simulink model "Fuzzy_BLDC"  (R2023a)
settings: Solver=ode1  StartTime=0.0  StopTime=50  FixedStep=0.1  RelTol=1e-3
values from neighbouring files (symbols this model uses):
  command_values = 0:6    [GenerateLUT_Fuzzy.m]
  error_pitch_values = -90:5:90    [GenerateLUT_Fuzzy.m]
  error_yaw_values = -180:5:180    [GenerateLUT_Fuzzy.m]
  fuzzy_lut_pitch = zeros(length(error_pitch_values), length(var_error_pitch_values), length(command_values), 2)    [GenerateLUT_Fuzzy.m]
  fuzzy_lut_yaw = zeros(length(error_yaw_values), length(var_error_yaw_values), length(command_values), 2)    [GenerateLUT_Fuzzy.m]
  var_error_pitch_values = -30:5:30    [GenerateLUT_Fuzzy.m]
  var_error_yaw_values = -50:5:50    [GenerateLUT_Fuzzy.m]
settings Model: Creator=yafhers  LastModifiedBy=yafhers
settings OptimizationCC: BlockReduction=off  ConditionallyExecuteInputs=off  DefaultParameterBehavior=Inlined  EnhancedBackFolding=on  PassReuseOutputArgsAs=Individual arguments  ZeroExternalMemoryAtStartup=off  ZeroInternalMemoryAtStartup=off  OptimizeBlockOrder=speed  DifferentSizesBufferReuse=on  OptimizationCustomize=off  EfficientTunableParamExpr=on
settings DebuggingCC: ParameterTunabilityLossMsg=error
settings SFSimCC: MATLABDynamicMemAlloc=off  SimTargetLang=C++
settings RTWCC: Description=Embedded Coder  SystemTargetFile=ert.tlc  TemplateMakefile=ert_default_tmf
settings CodeAppCC: ForceParamTrailComments=on  IgnoreCustomStorageClasses=off  OperatorAnnotations=on  SimulinkDataObjDesc=on  SFDataObjDesc=on  InsertBlockDesc=on
settings ERTTargetCC: TargetLangStandard=C99 (ISO)  GenerateSampleERTMain=on  InlinedParameterPlacement=NonHierarchical  ERTCustomFileTemplate=example_file_process.tlc

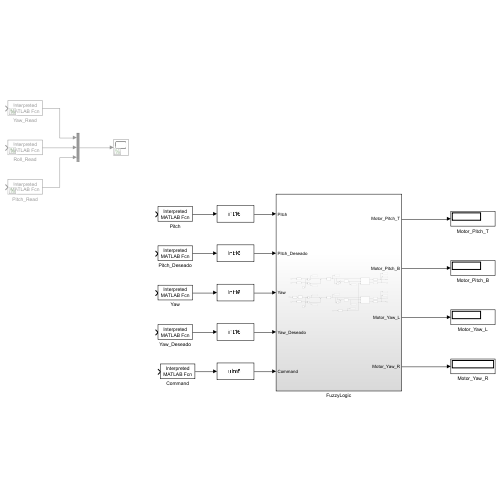
[thumbnail: Simulink's stored preview of the top-level diagram]
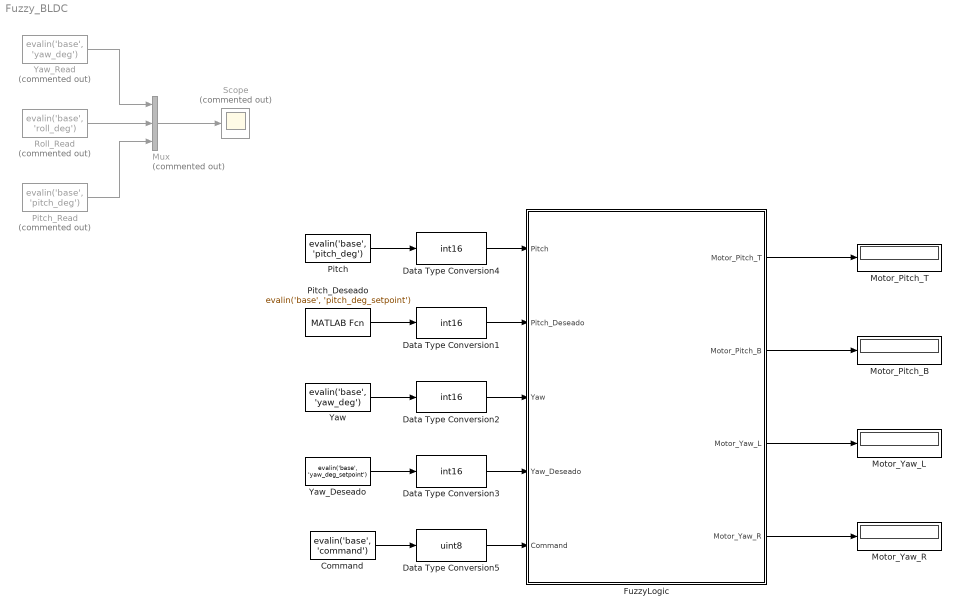
== system Fuzzy_BLDC ==
  Command : MATLABFcn  MATLABFcn=evalin('base', 'command')  OutputDimensions=1
  Data Type Conversion{1..4} (4 alike) : DataTypeConversion  OutDataTypeStr=int16  SaturateOnIntegerOverflow=off  RndMeth=Floor
  Data Type Conversion5 : DataTypeConversion  OutDataTypeStr=uint8  SaturateOnIntegerOverflow=off  RndMeth=Floor
  FuzzyLogic : Subsystem
  Motor_Pitch_B : Display
  Motor_Pitch_T : Display
  Motor_Yaw_L : Display
  Motor_Yaw_R : Display
  Mux : Mux  Commented=on  Inputs=3
  Pitch : MATLABFcn  MATLABFcn=evalin('base', 'pitch_deg')  OutputDimensions=1
  Pitch_Deseado : MATLABFcn  MATLABFcn=evalin('base', 'pitch_deg_setpoint')  OutputDimensions=1
  Pitch_Read : MATLABFcn  Commented=on  MATLABFcn=evalin('base', 'pitch_deg')  OutputDimensions=1  OutputSignalType=real
  Roll_Read : MATLABFcn  Commented=on  MATLABFcn=evalin('base', 'roll_deg')  OutputDimensions=1  OutputSignalType=real
  Scope : Scope  Commented=on
  Yaw : MATLABFcn  MATLABFcn=evalin('base', 'yaw_deg')  OutputDimensions=1
  Yaw_Deseado : MATLABFcn  MATLABFcn=evalin('base', 'yaw_deg_setpoint')  OutputDimensions=1
  Yaw_Read : MATLABFcn  Commented=on  MATLABFcn=evalin('base', 'yaw_deg')  OutputDimensions=1  OutputSignalType=real
  wires:
  Roll_Read/1 -> Mux/2
  Yaw_Read/1 -> Mux/1
  Pitch_Read/1 -> Mux/3
  Mux/1 -> Scope/1
  FuzzyLogic/2(Motor_Pitch_B) -> Motor_Pitch_B/1
  FuzzyLogic/1(Motor_Pitch_T) -> Motor_Pitch_T/1
  FuzzyLogic/3(Motor_Yaw_L) -> Motor_Yaw_L/1
  FuzzyLogic/4(Motor_Yaw_R) -> Motor_Yaw_R/1
  Command/1 -> Data Type Conversion5/1
  Data Type Conversion5/1 -> FuzzyLogic/5(Command)
  Pitch/1 -> Data Type Conversion4/1
  Data Type Conversion4/1 -> FuzzyLogic/1(Pitch)
  Pitch_Deseado/1 -> Data Type Conversion1/1
  Data Type Conversion1/1 -> FuzzyLogic/2(Pitch_Deseado)
  Yaw/1 -> Data Type Conversion2/1
  Data Type Conversion2/1 -> FuzzyLogic/3(Yaw)
  Yaw_Deseado/1 -> Data Type Conversion3/1
  Data Type Conversion3/1 -> FuzzyLogic/4(Yaw_Deseado)

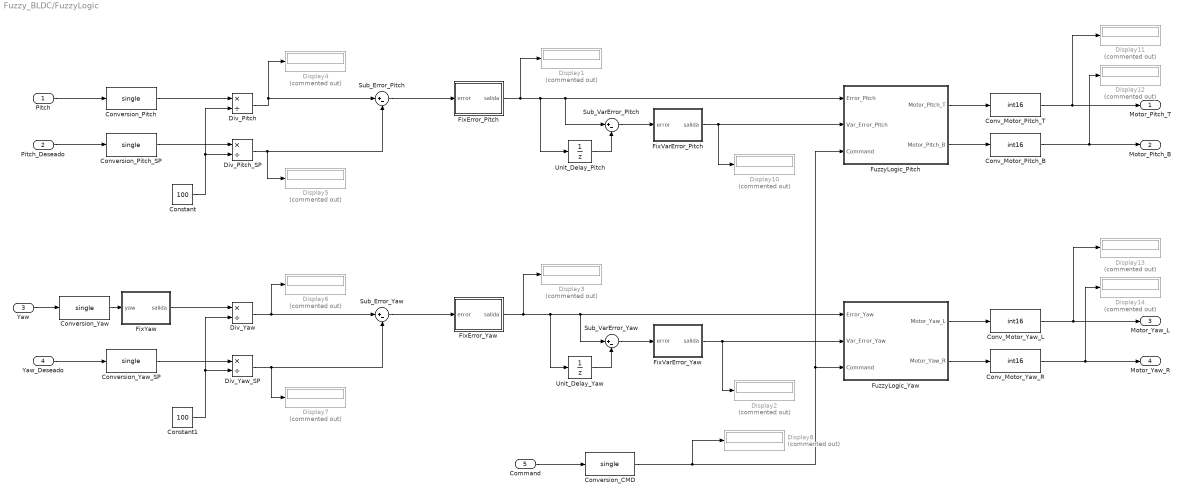
== system Fuzzy_BLDC/FuzzyLogic ==
  Pitch : Inport  OutDataTypeStr=int16
  Pitch_Deseado : Inport  Port=2  OutDataTypeStr=int16
  Yaw : Inport  Port=3  OutDataTypeStr=int16
  Yaw_Deseado : Inport  Port=4  OutDataTypeStr=int16
  Command : Inport  Port=5  OutDataTypeStr=uint8
  Constant : Constant  Value=100  OutDataTypeStr=single
  Constant1 : Constant  Value=100  OutDataTypeStr=single
  Conv_Motor_Pitch_B : DataTypeConversion  OutDataTypeStr=int16  SaturateOnIntegerOverflow=off  RndMeth=Floor
  Conv_Motor_Pitch_T : DataTypeConversion  OutDataTypeStr=int16  SaturateOnIntegerOverflow=off  RndMeth=Floor
  Conv_Motor_Yaw_L : DataTypeConversion  OutDataTypeStr=int16  SaturateOnIntegerOverflow=off  RndMeth=Floor
  Conv_Motor_Yaw_R : DataTypeConversion  OutDataTypeStr=int16  SaturateOnIntegerOverflow=off  RndMeth=Floor
  Conversion_CMD : DataTypeConversion  OutDataTypeStr=single  SaturateOnIntegerOverflow=off  RndMeth=Floor
  Conversion_Pitch : DataTypeConversion  OutDataTypeStr=single  SaturateOnIntegerOverflow=off  RndMeth=Floor
  Conversion_Pitch_SP : DataTypeConversion  OutDataTypeStr=single  SaturateOnIntegerOverflow=off  RndMeth=Floor
  Conversion_Yaw : DataTypeConversion  OutDataTypeStr=single  SaturateOnIntegerOverflow=off  RndMeth=Floor
  Conversion_Yaw_SP : DataTypeConversion  OutDataTypeStr=single  SaturateOnIntegerOverflow=off  RndMeth=Floor
  Display{1..8,10..14} (13 alike) : Display  Commented=on
  Div_Pitch : Product  Inputs=*/  OutDataTypeStr=single
  Div_Pitch_SP : Product  Inputs=*/  OutDataTypeStr=single
  Div_Yaw : Product  Inputs=*/  OutDataTypeStr=single
  Div_Yaw_SP : Product  Inputs=*/  OutDataTypeStr=single
  FixError_Pitch : MATLAB Function  TreatAsAtomicUnit=on
  FixError_Yaw : MATLAB Function  TreatAsAtomicUnit=on
  FixVarError_Pitch : MATLAB Function  TreatAsAtomicUnit=on
  FixVarError_Yaw : MATLAB Function  TreatAsAtomicUnit=on
  FixYaw : MATLAB Function  TreatAsAtomicUnit=on
  FuzzyLogic_Pitch : Subsystem
  FuzzyLogic_Yaw : Subsystem
  Sub_Error_Pitch : Sum  Inputs=|+-
  Sub_Error_Yaw : Sum  Inputs=|+-
  Sub_VarError_Pitch : Sum  Inputs=|+-
  Sub_VarError_Yaw : Sum  Inputs=|+-
  Unit_Delay_Pitch : UnitDelay  SampleTime=-1  HasFrameUpgradeWarning=on
  Unit_Delay_Yaw : UnitDelay  SampleTime=-1  HasFrameUpgradeWarning=on
  Motor_Pitch_T : Outport  OutDataTypeStr=int16
  Motor_Pitch_B : Outport  Port=2  OutDataTypeStr=int16
  Motor_Yaw_L : Outport  Port=3  OutDataTypeStr=int16
  Motor_Yaw_R : Outport  Port=4  OutDataTypeStr=int16
  wires:
  Unit_Delay_Pitch/1 -> Sub_VarError_Pitch/2
  Unit_Delay_Yaw/1 -> Sub_VarError_Yaw/2
  Yaw/1 -> Conversion_Yaw/1
  Pitch/1 -> Conversion_Pitch/1
  Pitch_Deseado/1 -> Conversion_Pitch_SP/1
  Command/1 -> Conversion_CMD/1
  Conversion_CMD/1 -> FuzzyLogic_Yaw/3(Command), FuzzyLogic_Pitch/3(Command), Display8/1
  Conversion_Pitch/1 -> Div_Pitch/1
  Conversion_Pitch_SP/1 -> Div_Pitch_SP/1
  Constant/1 -> Div_Pitch_SP/2, Div_Pitch/2
  Div_Pitch/1 -> Display4/1, Sub_Error_Pitch/1
  Div_Pitch_SP/1 -> Display5/1, Sub_Error_Pitch/2
  Constant1/1 -> Div_Yaw_SP/2, Div_Yaw/2
  Conversion_Yaw_SP/1 -> Div_Yaw_SP/1
  Div_Yaw_SP/1 -> Display7/1, Sub_Error_Yaw/2
  Yaw_Deseado/1 -> Conversion_Yaw_SP/1
  Sub_Error_Yaw/1 -> FixError_Yaw/1(error)
  Sub_Error_Pitch/1 -> FixError_Pitch/1(error)
  FixError_Yaw/1(salida) -> Display3/1, Unit_Delay_Yaw/1, Sub_VarError_Yaw/1, FuzzyLogic_Yaw/1(Error_Yaw)
  FixError_Pitch/1(salida) -> FuzzyLogic_Pitch/1(Error_Pitch), Sub_VarError_Pitch/1, Unit_Delay_Pitch/1, Display1/1
  FuzzyLogic_Pitch/1(Motor_Pitch_T) -> Conv_Motor_Pitch_T/1
  FuzzyLogic_Pitch/2(Motor_Pitch_B) -> Conv_Motor_Pitch_B/1
  FuzzyLogic_Yaw/2(Motor_Yaw_R) -> Conv_Motor_Yaw_R/1
  FuzzyLogic_Yaw/1(Motor_Yaw_L) -> Conv_Motor_Yaw_L/1
  Conv_Motor_Yaw_L/1 -> Display13/1, Motor_Yaw_L/1
  Conv_Motor_Yaw_R/1 -> Display14/1, Motor_Yaw_R/1
  Conv_Motor_Pitch_T/1 -> Display11/1, Motor_Pitch_T/1
  Conv_Motor_Pitch_B/1 -> Display12/1, Motor_Pitch_B/1
  Div_Yaw/1 -> Display6/1, Sub_Error_Yaw/1
  Conversion_Yaw/1 -> FixYaw/1(yaw)
  FixYaw/1(salida) -> Div_Yaw/1
  Sub_VarError_Pitch/1 -> FixVarError_Pitch/1(error)
  FixVarError_Pitch/1(salida) -> Display10/1, FuzzyLogic_Pitch/2(Var_Error_Pitch)
  Sub_VarError_Yaw/1 -> FixVarError_Yaw/1(error)
  FixVarError_Yaw/1(salida) -> Display2/1, FuzzyLogic_Yaw/2(Var_Error_Yaw)

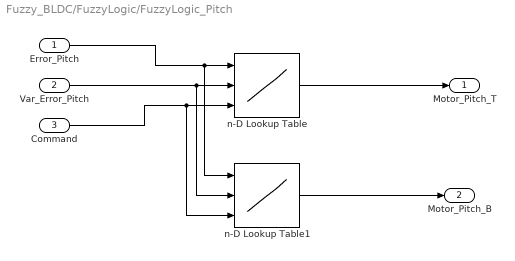
== system Fuzzy_BLDC/FuzzyLogic/FuzzyLogic_Pitch ==
  Error_Pitch : Inport
  Var_Error_Pitch : Inport  Port=2
  Command : Inport  Port=3
  n-D Lookup Table : Lookup_n-D  NumberOfTableDimensions=3  LookupTableObject=''  BreakpointsForDimension1=error_pitch_values  BreakpointsForDimension2=var_error_pitch_values  BreakpointsForDimension3=command_values  BreakpointsForDimension1FirstPoint=10  BreakpointsForDimension2FirstPoint=10  BreakpointsForDimension1Spacing=12  BreakpointsForDimension2Spacing=12  IndexSearchMethod=Evenly spaced points  Table=fuzzy_lut_pitch(:,:,:,1)  InterpMethod=Flat  DiagnosticForOutOfRangeInput=Error  InternalRulePriority=Speed  RndMeth=Simplest
      settings: InputPortMap=u0,u1,u2
  n-D Lookup Table1 : Lookup_n-D  NumberOfTableDimensions=3  LookupTableObject=''  BreakpointsForDimension1=error_pitch_values  BreakpointsForDimension2=var_error_pitch_values  BreakpointsForDimension3=command_values  BreakpointsForDimension1FirstPoint=10  BreakpointsForDimension2FirstPoint=10  BreakpointsForDimension1Spacing=12  BreakpointsForDimension2Spacing=12  IndexSearchMethod=Evenly spaced points  Table=fuzzy_lut_pitch(:,:,:,2)  InterpMethod=Flat  DiagnosticForOutOfRangeInput=Error  InternalRulePriority=Speed  RndMeth=Simplest
      settings: InputPortMap=u0,u1,u2
  Motor_Pitch_T : Outport
  Motor_Pitch_B : Outport  Port=2
  wires:
  n-D Lookup Table1/1 -> Motor_Pitch_B/1
  n-D Lookup Table/1 -> Motor_Pitch_T/1
  Error_Pitch/1 -> n-D Lookup Table/1, n-D Lookup Table1/1
  Var_Error_Pitch/1 -> n-D Lookup Table/2, n-D Lookup Table1/2
  Command/1 -> n-D Lookup Table/3, n-D Lookup Table1/3

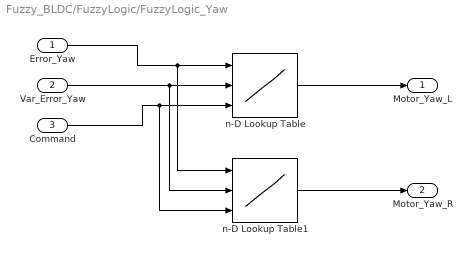
== system Fuzzy_BLDC/FuzzyLogic/FuzzyLogic_Yaw ==
  Error_Yaw : Inport  OutDataTypeStr=single
  Var_Error_Yaw : Inport  Port=2  OutDataTypeStr=single
  Command : Inport  Port=3  OutDataTypeStr=single
  n-D Lookup Table : Lookup_n-D  NumberOfTableDimensions=3  LookupTableObject=''  BreakpointsForDimension1=error_yaw_values  BreakpointsForDimension2=var_error_yaw_values  BreakpointsForDimension3=command_values  BreakpointsForDimension1FirstPoint=10  BreakpointsForDimension2FirstPoint=10  BreakpointsForDimension1Spacing=12  BreakpointsForDimension2Spacing=12  BreakpointsForDimension1DataTypeStr=single  BreakpointsForDimension2DataTypeStr=single  BreakpointsForDimension3DataTypeStr=single  IndexSearchMethod=Evenly spaced points  Table=fuzzy_lut_yaw(:,:,:,1)  TableDataTypeStr=single  InterpMethod=Flat  DiagnosticForOutOfRangeInput=Error  InternalRulePriority=Speed  OutDataTypeStr=single  RndMeth=Simplest
      settings: InputPortMap=u0,u1,u2
  n-D Lookup Table1 : Lookup_n-D  NumberOfTableDimensions=3  LookupTableObject=''  BreakpointsForDimension1=error_yaw_values  BreakpointsForDimension2=var_error_yaw_values  BreakpointsForDimension3=command_values  BreakpointsForDimension1FirstPoint=10  BreakpointsForDimension2FirstPoint=10  BreakpointsForDimension1Spacing=12  BreakpointsForDimension2Spacing=12  BreakpointsForDimension1DataTypeStr=single  BreakpointsForDimension2DataTypeStr=single  BreakpointsForDimension3DataTypeStr=single  IndexSearchMethod=Evenly spaced points  Table=fuzzy_lut_yaw(:,:,:,2)  TableDataTypeStr=single  InterpMethod=Flat  DiagnosticForOutOfRangeInput=Error  InternalRulePriority=Speed  OutDataTypeStr=single  RndMeth=Simplest
      settings: InputPortMap=u0,u1,u2
  Motor_Yaw_L : Outport
  Motor_Yaw_R : Outport  Port=2
  wires:
  n-D Lookup Table/1 -> Motor_Yaw_L/1
  Error_Yaw/1 -> n-D Lookup Table1/1, n-D Lookup Table/1
  Var_Error_Yaw/1 -> n-D Lookup Table1/2, n-D Lookup Table/2
  Command/1 -> n-D Lookup Table1/3, n-D Lookup Table/3
  n-D Lookup Table1/1 -> Motor_Yaw_R/1

== matlab function Fuzzy_BLDC/FuzzyLogic/FixError_Pitch ==
  data: error input; salida output
function salida = corrige_error(error)
    if error > 180
        salida = error - 360;
    elseif error < -180
        salida = error + 360;
    else
        salida = error;
    end

    salida = round(salida / 5) * 5;
end

== matlab function Fuzzy_BLDC/FuzzyLogic/FixYaw ==
  data: yaw input; salida output
function salida = corrige_yaw(yaw)
    if yaw < 0 
        salida = single(0.0);
    else
        salida = yaw;
    end
end

== matlab function Fuzzy_BLDC/FuzzyLogic/FixVarError_Pitch ==
  data: error input; salida output
function salida = corrige_error(error)
    if error > 30
        salida = single(30.0);
    elseif error < -30
        salida = single(-30.0);
    else
        salida = error;
    end

    salida = round(salida / 5) * 5;
end

== matlab function Fuzzy_BLDC/FuzzyLogic/FixVarError_Yaw ==
  data: error input; salida output
function salida = corrige_error(error)
    if error > 50
        salida = single(30.0);
    elseif error < -50
        salida = single(-30.0);
    else
        salida = error;
    end

    salida = round(salida / 5) * 5;
end

== matlab function Fuzzy_BLDC/FuzzyLogic/FixError_Yaw ==
  data: error input; salida output
function salida = corrige_error(error)
    if error > 180
        salida = (error - 360);
    elseif error < -180
        salida = (error + 360);
    else
        salida = error;
    end

    salida = round(salida / 5) * 5;
end
